simulink model "DP2_simlink"  (R2024b)
settings: Solver=FixedStepDiscrete  StartTime=0.0  StopTime=11380  FixedStep=1  RelTol=1e-3
undefined symbols (not defined in the file or in its folder): Ad, Bd, Cd, Dd, Pss, R_inv
settings Model: Creator=zalak  LastModifiedBy=zalak

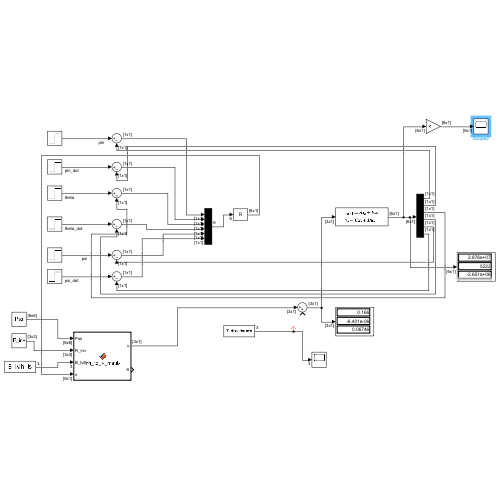
[thumbnail: Simulink's stored preview of the top-level diagram]
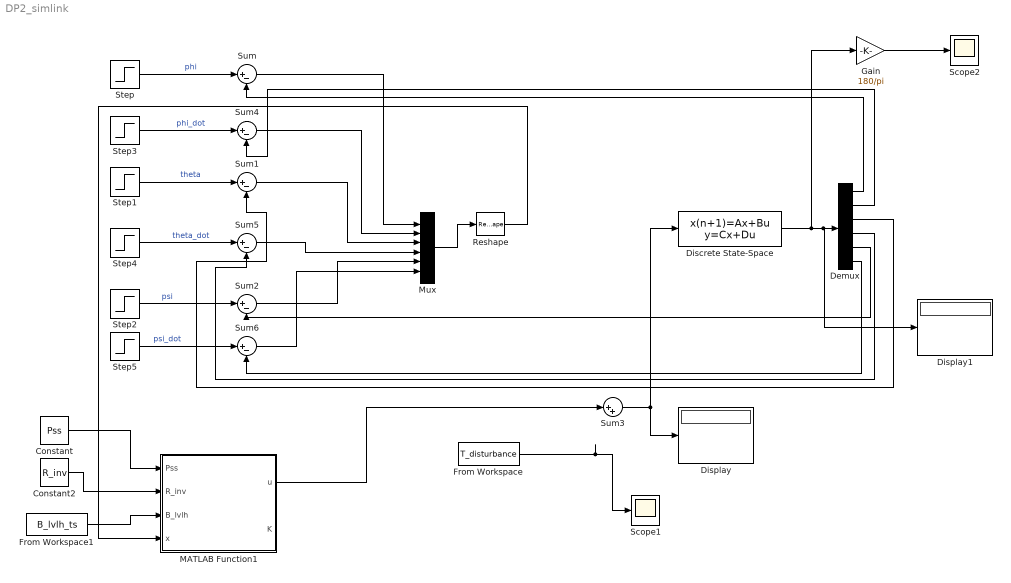
== system DP2_simlink ==
  Constant : Constant  Value=Pss
  Constant2 : Constant  Value=R_inv
  Demux : Demux  Outputs=6
  Discrete State-Space : DiscreteStateSpace  A=Ad  B=Bd  C=Cd  D=Dd  InitialCondition=[2*pi/180, 0, 2*pi/180, 0, 2*pi/180, 0]
  Display : Display
  Display1 : Display
  From Workspace : FromWorkspace  VariableName=T_disturbance
  From Workspace1 : FromWorkspace  VariableName=B_lvlh_ts  SampleTime=10
  Gain : Gain  Gain=180/pi
  MATLAB Function1 : MATLAB Function  TreatAsAtomicUnit=on
  Mux : Mux  Inputs=6
  Reshape : Reshape  OutputDimensionality=Customize  OutputDimensions=[6,1]
  Scope1 : Scope
  Scope2 : Scope
  Step{,1..5} (6 alike) : Step  Time=0  After=0  SampleTime=10
  Sum{,1..2,4..6} (6 alike) : Sum  Inputs=|+-
  Sum3 : Sum  Inputs=|++
  wires:
  Demux/1 -> Sum/2
  Step/1 -> Sum/1  "phi"
  Step2/1 -> Sum2/1  "psi"
  Sum/1 -> Mux/1
  Sum1/1 -> Mux/3
  Step1/1 -> Sum1/1  "theta"
  Sum2/1 -> Mux/5
  Mux/1 -> Reshape/1
  Reshape/1 -> MATLAB Function1/4(x)
  MATLAB Function1/1(u) -> Sum3/1
  Sum3/1 -> Display/1, Discrete State-Space/1
  From Workspace/1 -> Scope1/1
  Gain/1 -> Scope2/1
  From Workspace1/1 -> MATLAB Function1/3(B_lvlh)
  Constant/1 -> MATLAB Function1/1(Pss)
  Constant2/1 -> MATLAB Function1/2(R_inv)
  Discrete State-Space/1 -> Gain/1, Display1/1, Demux/1
  Step3/1 -> Sum4/1  "phi_dot"
  Demux/3 -> Sum1/2
  Demux/5 -> Sum2/2
  Demux/2 -> Sum4/2
  Sum4/1 -> Mux/2
  Step4/1 -> Sum5/1  "theta_dot"
  Demux/4 -> Sum5/2
  Sum5/1 -> Mux/4
  Sum6/1 -> Mux/6
  Demux/6 -> Sum6/2
  Step5/1 -> Sum6/1  "psi_dot"

== matlab function DP2_simlink/MATLAB Function1 ==
  data: Pss input; R_inv input; B_lvlh input; x input; u output; K output
function [u, K] = lvlh_to_K_matrix(Pss, R_inv, B_lvlh, x)
% Inputs:  Pss   (6×6) constant — from workspace
%          R_inv (3×3) constant — from workspace
%          B_lvlh (3×1) current field in LVLH — from From Workspace
%          x     (6×1) current state — from plant output
%
% No P feedback loop needed — Pss is constant

Ix = 0.00333;  Iy = 0.01020;  Iz = 0.01020;
m_max   = 0.166;    % A·m²
alpha0  = 10.0;     % gain scalar — increase for faster response at small errors

%% LVLH → body
phi = x(1);  theta = x(3);  psi = x(5);

Rx = [1, 0, 0; 0, cos(phi), sin(phi); 0, -sin(phi), cos(phi)];
Ry = [cos(theta), 0, -sin(theta); 0, 1, 0; sin(theta), 0, cos(theta)];
Rz = [cos(psi), sin(psi), 0; -sin(psi), cos(psi), 0; 0, 0, 1];

B_body = Rz * Ry * Rx * B_lvlh(:);

%% Build B_tv
Bx = B_body(1);  By = B_body(2);  Bz = B_body(3);

B_cross = [0, Bz, -By; 
          -Bz, 0, Bx; 
           By, -Bx, 0];

B_tv = zeros(6,3);
B_tv(2,:) = B_cross(1,:) / Ix;
B_tv(4,:) = B_cross(3,:) / Iz;
B_tv(6,:) = B_cross(2,:) / Iy;

%% Gain — Pss is constant, only B_tv varies
K     = alpha0 * R_inv * (B_tv' * Pss);   % (3×6)
u_nom = -K * x;                            % (3×1)

%% Proportional saturation (Psiaki eq 2b/2c)
beta = max(abs(u_nom) / m_max);   % scalar worst-case ratio
if beta <= 1
    u = u_nom;
else
    u = u_nom / beta;             % scale all axes together — preserves direction
end
